simulink model "proces"  (R2023a)
settings: Solver=VariableStepAuto  StartTime=0.0  StopTime=10.0  RelTol=1e-3
values from neighbouring files (symbols this model uses):
  Ts = 0.1    [all_signals.m]    (also in cutting_signals.m; get_outputs.m; main_3.m; noise.m)
libraries: PoKeysIOInterface x1
settings Model: Creator=64190198  LastModifiedBy=Gasper
settings SolverCC: AlgebraicLoopSolver=TrustRegion
settings DebuggingCC: UnconnectedInputMsg=warning  UnconnectedOutputMsg=warning  UnconnectedLineMsg=warning
settings ModelReferenceCC: EnableRefExpFcnMdlSchedulingChecks=on
settings RTWCC: DLArmComputeVersion=19.05

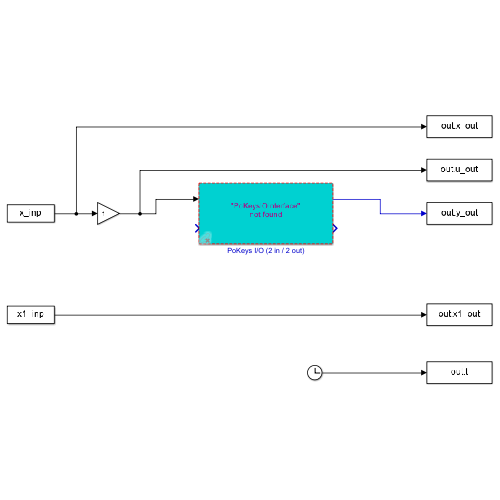
[thumbnail: Simulink's stored preview of the top-level diagram]
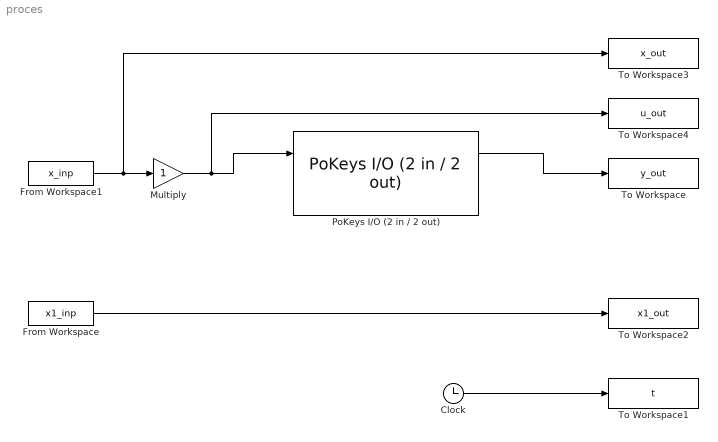
== system proces ==
  Clock : Clock
  From Workspace : FromWorkspace  VariableName=x1_inp  SampleTime=Ts
  From Workspace1 : FromWorkspace  VariableName=x_inp  SampleTime=Ts
  Multiply : Gain
  PoKeys I/O (2 in / 2 out) : PoKeysIOInterface/PoKeys I//O (2 in // 2 out)  MaxPowerLimit=100.0  IOTs=Ts  IOSerial=500
  To Workspace : ToWorkspace  VariableName=y_out  SampleTime=Ts
  To Workspace1 : ToWorkspace  VariableName=t  SampleTime=Ts
  To Workspace2 : ToWorkspace  VariableName=x1_out  SaveFormat=Timeseries  SampleTime=-1
  To Workspace3 : ToWorkspace  VariableName=x_out  SaveFormat=Timeseries  SampleTime=-1
  To Workspace4 : ToWorkspace  VariableName=u_out  SaveFormat=Timeseries  SampleTime=-1
  wires:
  Clock/1 -> To Workspace1/1
  PoKeys I/O (2 in / 2 out)/1 -> To Workspace/1
  From Workspace/1 -> To Workspace2/1
  From Workspace1/1 -> To Workspace3/1, Multiply/1
  Multiply/1 -> To Workspace4/1, PoKeys I/O (2 in / 2 out)/1
